simulink model "Des_Model"  (R2016b)
settings: Solver=ode3  StartTime=0.0  StopTime=Inf  RelTol=1e-3  EnableMultiTasking=on
settings Model: Creator=admim  LastModifiedBy=silviobacci
settings DataIOCC: LimitDataPoints=on  SaveFormat=Array
settings OptimizationCC: DefaultParameterBehavior=Inlined  InlineInvariantSignals=on  MaxStackSize=64
settings DebuggingCC: SolverPrmCheckMsg=warning  ParameterTunabilityLossMsg=error  SFUnexpectedBacktrackingDiag=warning  SFNoUnconditionalDefaultTransitionDiag=warning  SFExecutionAtInitializationDiag=none
settings HardwareCC: ProdBitPerPointer=32  ProdBitPerSizeT=32  ProdBitPerPtrDiffT=32  ProdLargestAtomicFloat=None  ProdIntDivRoundTo=Undefined  ProdEndianess=Unspecified  ProdWordSize=32  ProdHWDeviceType=Generic->Unspecified (assume 32-bit Generic)
settings ModelReferenceCC: PropagateSignalLabelsOutOfModel=off
settings RTWCC: SystemTargetFile=ert.tlc  GenCodeOnly=on  TemplateMakefile=ert_default_tmf  Description=Embedded Coder
settings CodeAppCC: ForceParamTrailComments=on  IgnoreCustomStorageClasses=off  OperatorAnnotations=on  SimulinkDataObjDesc=on  SFDataObjDesc=on  MATLABFcnDesc=on  InsertBlockDesc=on  MATLABSourceComments=on
settings ERTTargetCC: TargetLangStandard=C99 (ISO)  MultiInstanceERTCode=on  CodeInterfacePackaging=Reusable function  InlinedParameterPlacement=NonHierarchical  MultiInstanceErrorCode=None  ERTCustomFileTemplate=example_file_process.tlc
settings ConfigComp: CovMetricSettings=dw  CovHtmlReporting=on  CovSaveCumulativeToWorkspaceVar=on  CovSaveSingleToWorkspaceVar=on  CovExternalEMLEnable=off  CovSFcnEnable=off

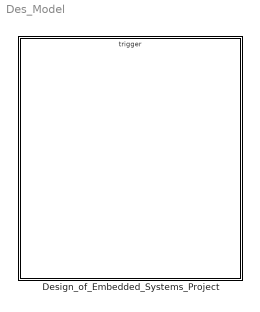
== system Des_Model ==
  Design_of_Embedded_Systems_Project : Stateflow chart  TreatAsAtomicUnit=on

== stateflow chart Des_Model/Design_of_Embedded_Systems_Project ==
  settings: executeAtInitialization=1
  state Car modes [parallel]
    settings: executionOrder=1
    state Obstacle_Avoiding
      en:
      turnLedOn();
      du:
      avoidObstacle();
      goToLineSearching = true;
    state Setup
      du:
      goStraight(T5);
      goToLineSearching = true;
      ex:
      turnLedOn();
      goToLineSearching = false;
    state Line_Following
      en:
      turnLedOff();
      obstacleFound = false;
      du:
      while(~obstacleFound) {
      followLine();
      obstacleFound = detectObstacle();
      }
    state Line_Searching
      en:
      keepMoving();
      lineFound = false;
      du:
      while(~lineFound) {
      lineFound = SearchLine();
      }
    Obstacle_Avoiding -> Line_Searching : [goToLineSearching == true]
    (default) -> Setup : [Turn on the car]
    Setup -> Line_Searching : [goToLineSearching == true]
    Line_Following -> Obstacle_Avoiding : [obstacleFound == true]
    Line_Searching -> Line_Following : [lineFound == true]
  events: ttick input EITHER_EDGE_EVENT
